simulink model "lr3"  (R2024a)
settings: Solver=ode23tb  StartTime=0.0  StopTime=0.4  MaxStep=1e-4  RelTol=1e-3
undefined symbols (not defined in the file or in its folder): angle_reg, D1, frequency, lagging, load, pulse, Source, Tran
libraries: spsThyristorLib x6, spsFourierLib x4, spsSeriesRLCBranchLib x4, spsVoltageMeasurementLib x4, spsACVoltageSourceLib x3, spsCurrentMeasurementLib x2, spsGroundLib x1, spsRMSLib x1, spsPLL3phLib x1, spsPulseGeneratorThyristor6PulseLib x1, spsThreePhaseVIMeasurementLib x1, sps_lib x1
settings Model: Creator=79532  LastModifiedBy=Руслан
settings SolverCC: ZeroCrossAlgorithm=Adaptive
settings DebuggingCC: IgnoredZcDiagnostic=none

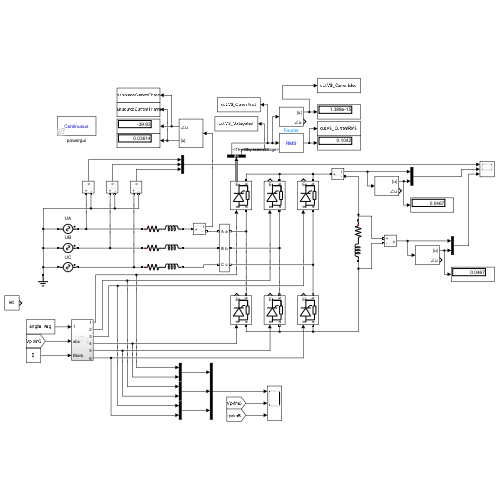
[thumbnail: Simulink's stored preview of the top-level diagram]
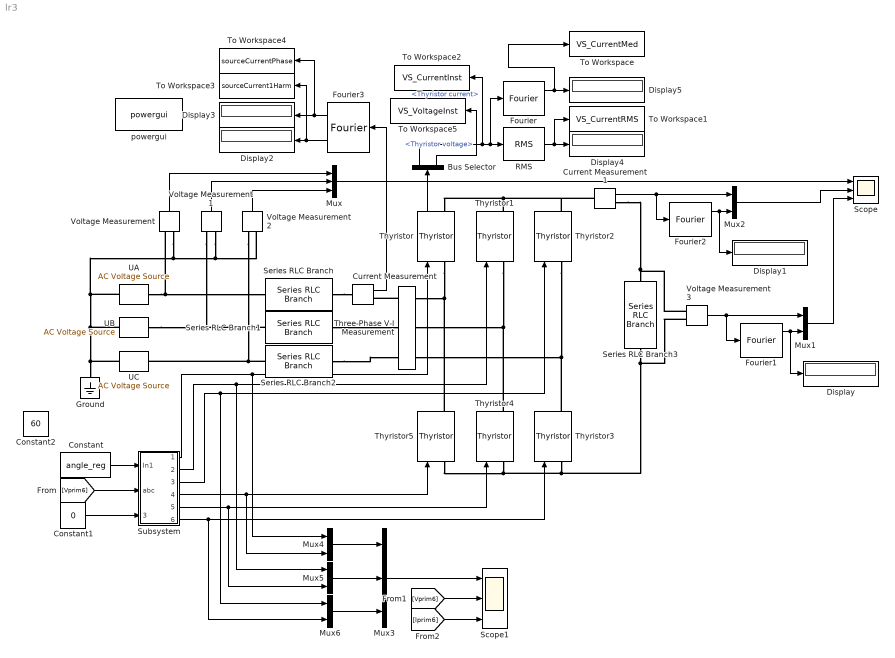
== system lr3 ==
  Bus Selector : BusSelector  OutputSignals=Thyristor current,Thyristor voltage
  Constant : Constant  Value=angle_reg
  Constant1 : Constant  Value=0
  Constant2 : Constant  Value=60
  Current Measurement : spsCurrentMeasurementLib/Current Measurement  PhasorSimulation=off  OutputType=Complex  PSBequivalent=0
  Current Measurement1 : spsCurrentMeasurementLib/Current Measurement  PhasorSimulation=off  OutputType=Complex  PSBequivalent=0
  Display{,1..5} (6 alike) : Display
  Fourier : spsFourierLib/Fourier  Freq=frequency*2  n=0  InInit=[0, 0]  Ts=0
  Fourier1 : spsFourierLib/Fourier  Freq=frequency*2  n=0  InInit=[0, 0]  Ts=0
  Fourier2 : spsFourierLib/Fourier  Freq=50  n=0  InInit=[0, 0]  Ts=0
  Fourier3 : spsFourierLib/Fourier  Freq=frequency  n=1  InInit=[0, 0]  Ts=0
  Ground : spsGroundLib/Ground  LConnTagsString=a
  Mux : Mux  Inputs=3
  Mux{1..2,4..6} (5 alike) : Mux  Inputs=2
  Mux3 : Mux  Inputs=3
  RMS : spsRMSLib/RMS  TrueRMS=on  Freq=frequency  RMSInit=0  Ts=0.0001
  Scope : Scope  NumInputPorts=3
  Scope1 : Scope  NumInputPorts=3
  Series RLC Branch : spsSeriesRLCBranchLib/Series RLC Branch  LConnTagsString=__new0  RConnTagsString=__new0  BranchType=RL  Resistance=Tran.Resistance  Inductance=Tran.Inductance  SetiL0=off  InitialCurrent=0  Capacitance=1e-6  Setx0=off  InitialVoltage=0  Measurements=None
  Series RLC Branch1 : spsSeriesRLCBranchLib/Series RLC Branch  LConnTagsString=__new0  RConnTagsString=__new0  BranchType=RL  Resistance=Tran.Resistance  Inductance=Tran.Inductance  SetiL0=off  InitialCurrent=0  Capacitance=1e-6  Setx0=off  InitialVoltage=0  Measurements=None
  Series RLC Branch2 : spsSeriesRLCBranchLib/Series RLC Branch  LConnTagsString=__new0  RConnTagsString=__new0  BranchType=RL  Resistance=Tran.Resistance  Inductance=Tran.Inductance  SetiL0=off  InitialCurrent=0  Capacitance=1e-6  Setx0=off  InitialVoltage=0  Measurements=None
  Series RLC Branch3 : spsSeriesRLCBranchLib/Series RLC Branch  LConnTagsString=__new0  RConnTagsString=__new0  BranchType=RL  Resistance=load.Res  Inductance=load.Ind  SetiL0=off  InitialCurrent=0  Capacitance=1e-6  Setx0=off  InitialVoltage=0  Measurements=None
  Subsystem : Subsystem
  Three-Phase V-I Measurement : spsThreePhaseVIMeasurementLib/Three-Phase V-I Measurement  VoltageMeasurement=phase-to-ground  SetLabelV=on  LabelV=Vprim6  Vpu=off  VpuLL=off  CurrentMeasurement=yes  SetLabelI=on  LabelI=Iprim6  Ipu=off  Pbase=100e6  Vbase=500e3  OutputType=Complex  PhasorSimulation=off  PSBequivalent=0
  Thyristor{,1..5} (6 alike) : spsThyristorLib/Thyristor  Ron=Thyr.ResistanceRon  Lon=0  Vf=Thyr.ForwVolt  IC=0  Rs=500  Cs=250e-9  Measurements=on
  To Workspace : ToWorkspace  VariableName=VS_CurrentMed  SaveFormat=Timeseries  SampleTime=-1
  To Workspace1 : ToWorkspace  VariableName=VS_CurrentRMS  SaveFormat=Timeseries  SampleTime=-1
  To Workspace2 : ToWorkspace  VariableName=VS_CurrentInst  SaveFormat=Timeseries  SampleTime=-1
  To Workspace3 : ToWorkspace  VariableName=sourceCurrent1Harm  SaveFormat=Timeseries  SampleTime=-1
      settings: Save2DSignal=2-D array (concatenate along first dimension)
  To Workspace4 : ToWorkspace  VariableName=sourceCurrentPhase  SaveFormat=Timeseries  SampleTime=-1
      settings: Save2DSignal=2-D array (concatenate along first dimension)
  To Workspace5 : ToWorkspace  VariableName=VS_VoltageInst  SaveFormat=Timeseries  SampleTime=-1
  UA : spsACVoltageSourceLib/AC Voltage Source  Amplitude=Source.VoltageAmplitude  Phase=0  Frequency=frequency  SampleTime=0  Measurements=None  BusType=swing  Pref=10e3  Qref=0  Qmin=-inf  Qmax=+inf
  UB : spsACVoltageSourceLib/AC Voltage Source  Amplitude=Source.VoltageAmplitude  Phase=240  Frequency=frequency  SampleTime=0  Measurements=None  BusType=swing  Pref=10e3  Qref=0  Qmin=-inf  Qmax=+inf
  UC : spsACVoltageSourceLib/AC Voltage Source  Amplitude=Source.VoltageAmplitude  Phase=120  Frequency=frequency  SampleTime=0  Measurements=None  BusType=swing  Pref=10e3  Qref=0  Qmin=-inf  Qmax=+inf
  Voltage Measurement{,1..3} (4 alike) : spsVoltageMeasurementLib/Voltage Measurement  PhasorSimulation=off  OutputType=Complex  PSBequivalent=0
  powergui : sps_lib/powergui  Priority=1  SimulationMode=Continuous  SampleTime=50e-6  frequency=60  Iterations=50  frequencyindice=50  Pbase=100e6  ErrMax=1e-4  UnitsV=kV  UnitsW=MW  buscounter=0  FunctionMessages=off  echomessages=off  EnableUseOfTLC=off  CurrentSourceSwitches=off  DisableSnubberDevices=off  DisableRonSwitches=off  DisableVfSwitches=off  DisplayEquations=off  AutomaticDiscreteSolvers=off  SolverType=Tustin/Backward Euler (TBE)  Interpol=off  ExternalGateDelay=off  methode=off  Ts=100  x0status=blocks  SPID=on  SwTol=0  HookPort=off  NonlinearTolerance=1e-4  nMaxIteration=100  ContinueOnMaxIteration=off  RestoreLinks=warning  ResistiveCurrentMeasurement=off  Frange=[0:2:500]  Ylog=off  Xlog=on  ShowGrid=off  save=off  variable=ZData  structure=0  ZoomFFT=off  StartTime=0.0  cycles=1  DisplayStyle=1  fundamental=60  FreqAxis=off  MaxFrequency=1000  frequencyindicesteady=1  RmsSteady=1  display=off
  wires:
  Voltage Measurement/1 -> Mux/1
  Voltage Measurement1/1 -> Mux/2
  Voltage Measurement2/1 -> Mux/3
  Current Measurement/1 -> Fourier3/1
  Fourier1/1 -> Display/1, Mux1/2
  Voltage Measurement3/1 -> Fourier1/1, Mux1/1
  Current Measurement1/1 -> Fourier2/1, Mux2/1
  Fourier2/1 -> Mux2/2, Display1/1
  Mux1/1 -> Scope/3
  Mux2/1 -> Scope/2
  Mux/1 -> Scope/1
  Fourier3/1 -> To Workspace3/1, Display2/1
  Fourier3/2 -> To Workspace4/1, Display3/1
  Thyristor/1 -> Bus Selector/1
  Bus Selector/1 -> To Workspace2/1, Fourier/1, RMS/1  "<Thyristor current>"
  RMS/1 -> To Workspace1/1, Display4/1
  Subsystem/1(Out1) -> Mux4/1, Thyristor/1
  Subsystem/2(Out2) -> Thyristor1/1, Mux5/1
  Subsystem/3(Out3) -> Thyristor2/1, Mux6/1
  Subsystem/4(Out4) -> Thyristor5/1, Mux4/2
  Subsystem/5(Out5) -> Thyristor4/1, Mux5/2
  Subsystem/6(Out6) -> Thyristor3/1, Mux6/2
  Mux4/1 -> Mux3/1
  Mux5/1 -> Mux3/2
  Mux6/1 -> Mux3/3
  Constant/1 -> Subsystem/1(In1)
  [Vprim6] -> Subsystem/2(abc)
  Constant1/1 -> Subsystem/3(Block)
  Mux3/1 -> Scope1/1
  [Vprim6] -> Scope1/2
  [Iprim6] -> Scope1/3
  Bus Selector/2 -> To Workspace5/1  "<Thyristor voltage>"
  Fourier/1 -> To Workspace/1, Display5/1
  connections:
  UA/LConn1 -- Voltage Measurement/LConn2 -- Voltage Measurement1/LConn2 -- Voltage Measurement2/LConn2 -- UB/LConn1 -- UC/LConn1 -- Ground/LConn1
  Voltage Measurement2/LConn1 -- Series RLC Branch2/LConn1 -- UC/RConn1
  UB/RConn1 -- Series RLC Branch1/LConn1 -- Voltage Measurement1/LConn1
  UA/RConn1 -- Voltage Measurement/LConn1 -- Series RLC Branch/LConn1
  Thyristor/LConn1 -- Thyristor5/RConn1 -- Three-Phase V-I Measurement/RConn1
  Three-Phase V-I Measurement/RConn2 -- Thyristor4/RConn1 -- Thyristor1/LConn1
  Three-Phase V-I Measurement/RConn3 -- Thyristor3/RConn1 -- Thyristor2/LConn1
  Series RLC Branch/RConn1 -- Current Measurement/LConn1
  Thyristor2/RConn1 -- Current Measurement1/LConn1 -- Thyristor/RConn1 -- Thyristor1/RConn1
  Series RLC Branch3/RConn1 -- Voltage Measurement3/LConn2 -- Thyristor3/LConn1 -- Thyristor5/LConn1 -- Thyristor4/LConn1
  Current Measurement1/RConn1 -- Voltage Measurement3/LConn1 -- Series RLC Branch3/LConn1
  Three-Phase V-I Measurement/LConn1 -- Current Measurement/RConn1
  Series RLC Branch1/RConn1 -- Three-Phase V-I Measurement/LConn2
  Series RLC Branch2/RConn1 -- Three-Phase V-I Measurement/LConn3

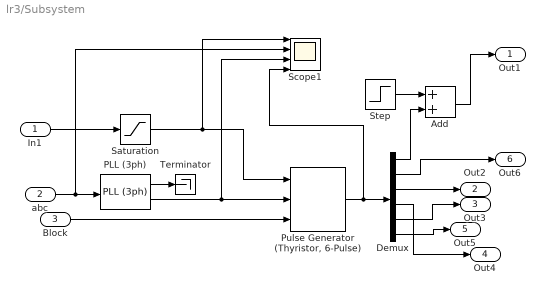
== system lr3/Subsystem ==
  In1 : Inport
  abc : Inport  Port=2
  Block : Inport  Port=3
  Add : Sum
  Demux : Demux  Outputs=6
  PLL (3ph) : spsPLL3phLib/PLL (3ph)  Fmin=45  Par_Init=[0, frequency]  ParK=[180, 3200, 1]  TcD=1e-4  MaxRateChangeFreq=12  FilterCutOffFreq=25  Ts=0.0001  AGC=on
  "Pulse Generator (Thyristor, 6-Pulse)" : spsPulseGeneratorThyristor6PulseLib/Pulse Generator (Thyristor, 6-Pulse)  GenType=6-pulse  Delta=D1 (lagging)  pwidth=5  Double_Pulse=off  Ts=0.0001
      settings: LibrarySourceBlock=|
      | sps_lib/Power Electronics/Power Electronics Control/Pulse Generator
      | (Thyristor, 6-Pulse)
  Saturation : Saturate  UpperLimit=120  LowerLimit=0
  Scope1 : Scope  NumInputPorts=4
  Step : Step  Time=1/frequency/2  Before=1  After=0  SampleTime=0.0001
  Terminator : Terminator
  Out1 : Outport
  Out2 : Outport  Port=2
  Out3 : Outport  Port=3
  Out4 : Outport  Port=4
  Out5 : Outport  Port=5
  Out6 : Outport  Port=6
  wires:
  abc/1 -> Scope1/2, PLL (3ph)/1
  Block/1 -> "Pulse Generator (Thyristor, 6-Pulse)"/3
  PLL (3ph)/1 -> Terminator/1
  Saturation/1 -> Scope1/1, "Pulse Generator (Thyristor, 6-Pulse)"/1
  "Pulse Generator (Thyristor, 6-Pulse)"/1 -> Scope1/4, Demux/1
  PLL (3ph)/2 -> Scope1/3, "Pulse Generator (Thyristor, 6-Pulse)"/2
  Demux/1 -> Add/2
  Step/1 -> Add/1
  In1/1 -> Saturation/1
  Add/1 -> Out1/1
  Demux/2 -> Out6/1
  Demux/3 -> Out2/1
  Demux/4 -> Out4/1
  Demux/5 -> Out3/1
  Demux/6 -> Out5/1
